simulink subsystem "HIB"  (R2023b)
settings: Solver=VariableStepAuto  StartTime=0.0  StopTime=10.0  RelTol=1e-3
libraries: simulink x1
settings Model: Creator=matat  LastModifiedBy=nickj

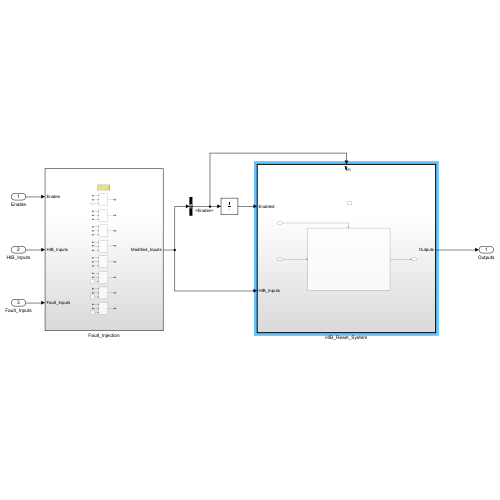
[thumbnail: Simulink's stored preview of the top-level diagram]
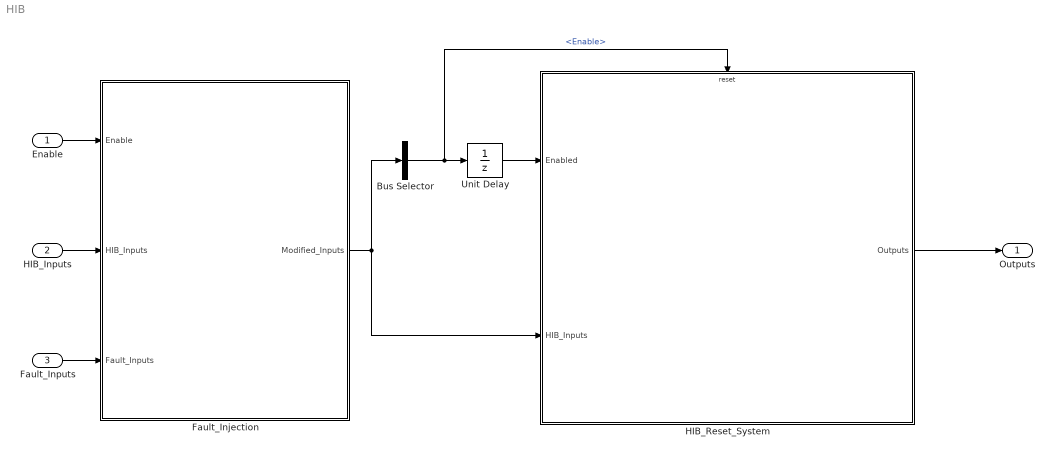
== system HIB ==
  Enable : Inport
  HIB_Inputs : Inport  Port=2
  Fault_Inputs : Inport  Port=3
  Bus Selector : BusSelector  OutputSignals=Enable
  Fault_Injection : Subsystem
  "HIB_Reset_System " : Subsystem  TreatAsAtomicUnit=on
  Unit Delay : UnitDelay  SampleTime=-1  HasFrameUpgradeWarning=on
  Outputs : Outport
  wires:
  Fault_Injection/1(Modified_Inputs) -> "HIB_Reset_System "/2(HIB_Inputs), Bus Selector/1
  "HIB_Reset_System "/1(Outputs) -> Outputs/1
  Unit Delay/1 -> "HIB_Reset_System "/1(Enabled)
  HIB_Inputs/1 -> Fault_Injection/2(HIB_Inputs)
  Fault_Inputs/1 -> Fault_Injection/3(Fault_Inputs)
  Enable/1 -> Fault_Injection/1(Enable)
  Bus Selector/1 -> Unit Delay/1, "HIB_Reset_System "/Reset  "<Enable>"

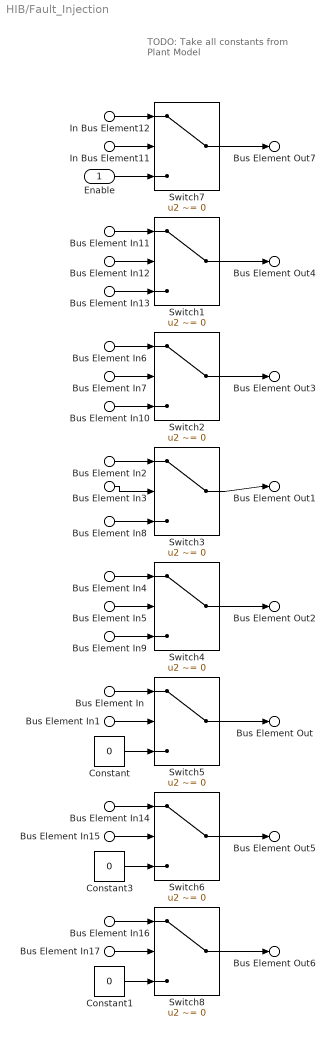
== system HIB/Fault_Injection ==
  note: TODO: Take all constants from Plant Model
  Enable : Inport
  Bus Element In8 : Inport  Port=2  PortName=HIB_Inputs  Element=Start
  Bus Element In9 : Inport  Port=2  PortName=HIB_Inputs  Element=Forward_EN
  Bus Element In10 : Inport  Port=2  PortName=HIB_Inputs  Element=Brake
  Bus Element In13 : Inport  Port=2  PortName=HIB_Inputs  Element=Throttle
  Bus Element In : Inport  Port=3  PortName=Fault_Inputs  Element=Comparison_Error_Count
  Bus Element In1 : Inport  Port=3  PortName=Fault_Inputs  Element=Override_Comparison_Error_Count
  Bus Element In2 : Inport  Port=3  PortName=Fault_Inputs  Element=Start
  Bus Element In4 : Inport  Port=3  PortName=Fault_Inputs  Element=Forward_EN
  Bus Element In3 : Inport  Port=3  PortName=Fault_Inputs  Element=Override_Start
  Bus Element In12 : Inport  Port=3  PortName=Fault_Inputs  Element=Override_Throttle
  Bus Element In7 : Inport  Port=3  PortName=Fault_Inputs  Element=Override_Brake
  Bus Element In5 : Inport  Port=3  PortName=Fault_Inputs  Element=Override_Forward_EN
  Bus Element In11 : Inport  Port=3  PortName=Fault_Inputs  Element=Throttle
  Bus Element In15 : Inport  Port=3  PortName=Fault_Inputs  Element=Override_Acceptable_Margin_Error_Count
  Bus Element In14 : Inport  Port=3  PortName=Fault_Inputs  Element=Acceptable_Margin_Error_Count
  Bus Element In17 : Inport  Port=3  PortName=Fault_Inputs  Element=Override_Precision_Margin_Error_Count
  Bus Element In16 : Inport  Port=3  PortName=Fault_Inputs  Element=Precision_Margin_Error_Count
  Bus Element In6 : Inport  Port=3  PortName=Fault_Inputs  Element=Brake
  In Bus Element12 : Inport  Port=3  PortName=Fault_Inputs  Element=HIB_EN
  In Bus Element11 : Inport  Port=3  PortName=Fault_Inputs  Element=Override_HIB_EN
  Constant : Constant  Value=0
  Constant1 : Constant  Value=0
  Constant3 : Constant  Value=0
  Switch{1..8} (8 alike) : Switch  Criteria=u2 ~= 0  SaturateOnIntegerOverflow=off  InputSameDT=off
  Bus Element Out : Outport  PortName=Modified_Inputs  Element=Errors.Comparison_Error_Count
  Bus Element Out5 : Outport  PortName=Modified_Inputs  Element=Errors.Acceptable_Margin_Error_Count
  Bus Element Out6 : Outport  PortName=Modified_Inputs  Element=Errors.Precision_Margin_Error_Count
  Bus Element Out4 : Outport  PortName=Modified_Inputs  Element=Throttle
  Bus Element Out3 : Outport  PortName=Modified_Inputs  Element=Brake
  Bus Element Out1 : Outport  PortName=Modified_Inputs  Element=Start
  Bus Element Out2 : Outport  PortName=Modified_Inputs  Element=Forward_EN
  Bus Element Out7 : Outport  PortName=Modified_Inputs  Element=Enable
  wires:
  Constant1/1 -> Switch8/3
  Switch5/1 -> Bus Element Out/1
  Constant3/1 -> Switch6/3
  Constant/1 -> Switch5/3
  Bus Element In13/1 -> Switch1/3
  Bus Element In/1 -> Switch5/1
  Bus Element In1/1 -> Switch5/2
  Bus Element In3/1 -> Switch3/2
  Bus Element In2/1 -> Switch3/1
  Switch3/1 -> Bus Element Out1/1
  Bus Element In5/1 -> Switch4/2
  Bus Element In4/1 -> Switch4/1
  Switch4/1 -> Bus Element Out2/1
  Bus Element In8/1 -> Switch3/3
  Bus Element In9/1 -> Switch4/3
  Bus Element In10/1 -> Switch2/3
  Switch2/1 -> Bus Element Out3/1
  Bus Element In6/1 -> Switch2/1
  Bus Element In7/1 -> Switch2/2
  Switch1/1 -> Bus Element Out4/1
  Bus Element In11/1 -> Switch1/1
  Bus Element In12/1 -> Switch1/2
  Switch6/1 -> Bus Element Out5/1
  Bus Element In14/1 -> Switch6/1
  Bus Element In15/1 -> Switch6/2
  Switch8/1 -> Bus Element Out6/1
  Bus Element In16/1 -> Switch8/1
  Bus Element In17/1 -> Switch8/2
  In Bus Element12/1 -> Switch7/1
  Switch7/1 -> Bus Element Out7/1
  In Bus Element11/1 -> Switch7/2
  Enable/1 -> Switch7/3

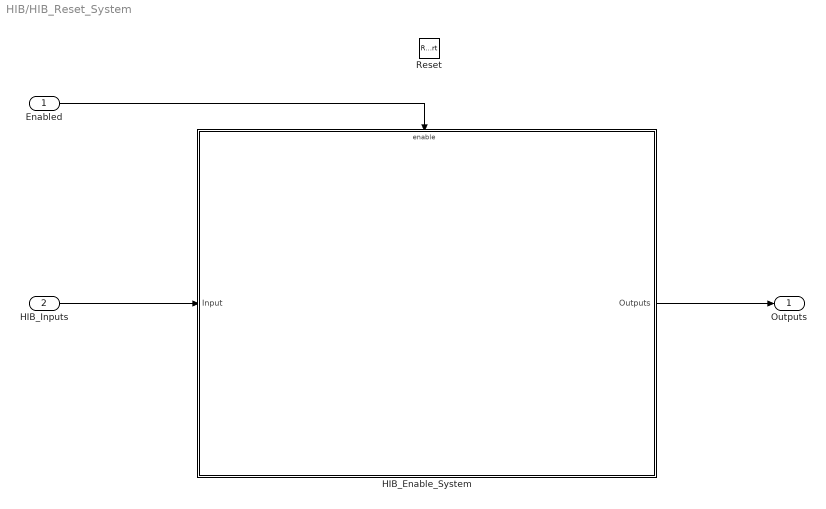
== system HIB/HIB_Reset_System  ==
  Enabled : Inport
  HIB_Inputs : Inport  Port=2
  Reset : ResetPort  DisableCoverage=on  ResetTriggerType=falling
  "HIB_Enable_System " : Subsystem  TreatAsAtomicUnit=on
  Outputs : Outport
  wires:
  "HIB_Enable_System "/1(Outputs) -> Outputs/1
  HIB_Inputs/1 -> "HIB_Enable_System "/1(Input)
  Enabled/1 -> "HIB_Enable_System "/Enable

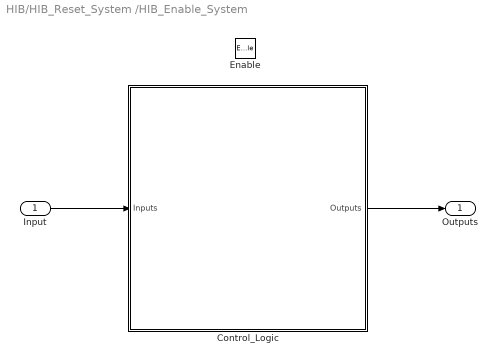
== system HIB/HIB_Reset_System /HIB_Enable_System  ==
  Input : Inport
  Enable : EnablePort  StatesWhenEnabling=reset
  Control_Logic : Subsystem
  Outputs : Outport
  wires:
  Control_Logic/1(Outputs) -> Outputs/1
  Input/1 -> Control_Logic/1(Inputs)

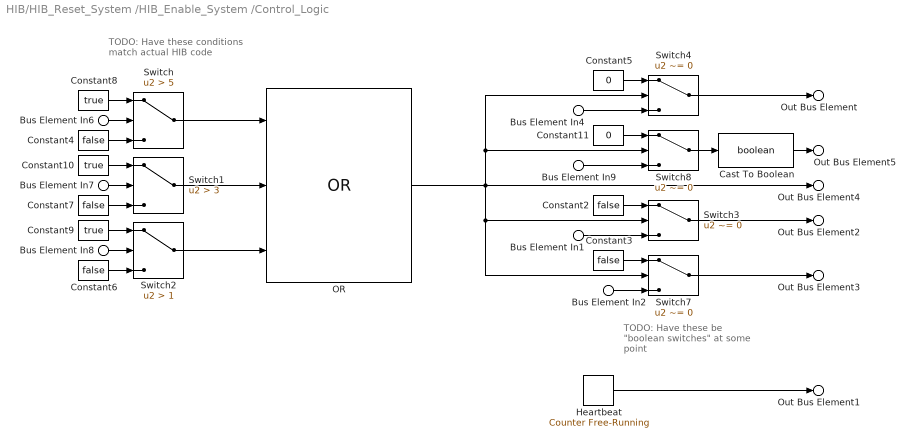
== system HIB/HIB_Reset_System /HIB_Enable_System /Control_Logic ==
  note: TODO: Have these conditions match actual HIB code
  note: TODO: Have these be "boolean switches" at some point
  Bus Element In2 : Inport  PortName=Inputs  Element=Start
  Bus Element In9 : Inport  PortName=Inputs  Element=Brake
  Bus Element In4 : Inport  PortName=Inputs  Element=Throttle
  Bus Element In6 : Inport  PortName=Inputs  Element=Errors.Acceptable_Margin_Error_Count
  Bus Element In7 : Inport  PortName=Inputs  Element=Errors.Precision_Margin_Error_Count
  Bus Element In8 : Inport  PortName=Inputs  Element=Errors.Comparison_Error_Count
  Bus Element In1 : Inport  PortName=Inputs  Element=Forward_EN
  Cast To Boolean : DataTypeConversion  OutDataTypeStr=boolean  SaturateOnIntegerOverflow=off  RndMeth=Floor
  Constant10 : Constant  Value=true
  Constant11 : Constant  Value=0
  Constant{2..4,6..7} (5 alike) : Constant  Value=false
  Constant5 : Constant  Value=0
  Constant8 : Constant  Value=true
  Constant9 : Constant  Value=true
  Heartbeat : simulink/Sources/Counter Free-Running  NumBits=32  tsamp=-1
  OR : Logic  Operator=OR  Inputs=3  IconShape=distinctive  AllPortsSameDT=off  OutDataTypeStr=boolean
  Switch : Switch  Criteria=u2 > Threshold  Threshold=5  SaturateOnIntegerOverflow=off  InputSameDT=off
  Switch1 : Switch  Criteria=u2 > Threshold  Threshold=3  SaturateOnIntegerOverflow=off  InputSameDT=off
  Switch2 : Switch  Criteria=u2 > Threshold  Threshold=1  SaturateOnIntegerOverflow=off  InputSameDT=off
  Switch{3..4,7..8} (4 alike) : Switch  Criteria=u2 ~= 0  SaturateOnIntegerOverflow=off  InputSameDT=off
  Out Bus Element2 : Outport  PortName=Outputs  Element=Forward_EN
  Out Bus Element3 : Outport  PortName=Outputs  Element=Start
  Out Bus Element : Outport  PortName=Outputs  Element=Throttle
  Out Bus Element4 : Outport  PortName=Outputs  Element=HIB_Comparison_Fault
  Out Bus Element5 : Outport  PortName=Outputs  Element=Brake
  Out Bus Element1 : Outport  PortName=Outputs  Element=HIB_Heartbeat
  wires:
  Heartbeat/1 -> Out Bus Element1/1
  OR/1 -> Switch3/2, Switch7/2, Switch4/2, Switch8/2, Out Bus Element4/1
  Bus Element In6/1 -> Switch/2
  Switch/1 -> OR/1
  Bus Element In7/1 -> Switch1/2
  Bus Element In8/1 -> Switch2/2
  Bus Element In4/1 -> Switch4/3
  Bus Element In1/1 -> Switch3/3
  Constant2/1 -> Switch3/1
  Constant3/1 -> Switch7/1
  Constant5/1 -> Switch4/1
  Switch4/1 -> Out Bus Element/1
  Switch3/1 -> Out Bus Element2/1
  Constant8/1 -> Switch/1
  Constant4/1 -> Switch/3
  Constant7/1 -> Switch1/3
  Constant10/1 -> Switch1/1
  Constant6/1 -> Switch2/3
  Constant9/1 -> Switch2/1
  Switch1/1 -> OR/2
  Switch2/1 -> OR/3
  Bus Element In9/1 -> Switch8/3
  Constant11/1 -> Switch8/1
  Bus Element In2/1 -> Switch7/3
  Switch7/1 -> Out Bus Element3/1
  Switch8/1 -> Cast To Boolean/1
  Cast To Boolean/1 -> Out Bus Element5/1
